simulink model "TailsitterSimModel_Trim"  (R2018b)
settings: Solver=ode23  StartTime=0  StopTime=1200  FixedStep=0.01  RelTol=1e-4  EnableMultiTasking=on
libraries: aerolibanimutils x1, tailsitter_lib x1, atmosphere_lib x1
settings Model: Creator=Yannic  LastModifiedBy=fabian
settings SolverCC: ZeroCrossControl=DisableAll  AlgebraicLoopSolver=LineSearch
settings DataIOCC: LimitDataPoints=on  SaveFormat=StructureWithTime
settings OptimizationCC: BlockReduction=off  DefaultParameterBehavior=Inlined  DefaultUnderspecifiedDataType=single  OptimizeBlockIOStorage=off  BufferReuse=off  GlobalBufferReuse=off  ExpressionFolding=off  LocalBlockOutputs=off  LifeSpan=inf  OptimizeDataStoreBuffers=off  BusAssignmentInplaceUpdate=off
settings DebuggingCC: AlgebraicLoopMsg=none  UnconnectedInputMsg=none  UnconnectedOutputMsg=none  UnconnectedLineMsg=none  AllowSymbolicDim=off  SFUnexpectedBacktrackingDiag=warning  SFNoUnconditionalDefaultTransitionDiag=warning  SFExecutionAtInitializationDiag=none
settings ModelReferenceCC: PropagateSignalLabelsOutOfModel=off
settings SFSimCC: SimUseLocalCustomCode=off
settings RTWCC: RTWUseLocalCustomCode=off
settings CodeAppCC: StateflowObjectComments=on
settings GRTTargetCC: TargetLangStandard=C89/C90 (ANSI)
settings ConfigComp: CovMetricSettings=dw  CovHtmlReporting=on  CovSaveCumulativeToWorkspaceVar=on  CovSaveSingleToWorkspaceVar=on  CovExternalEMLEnable=off

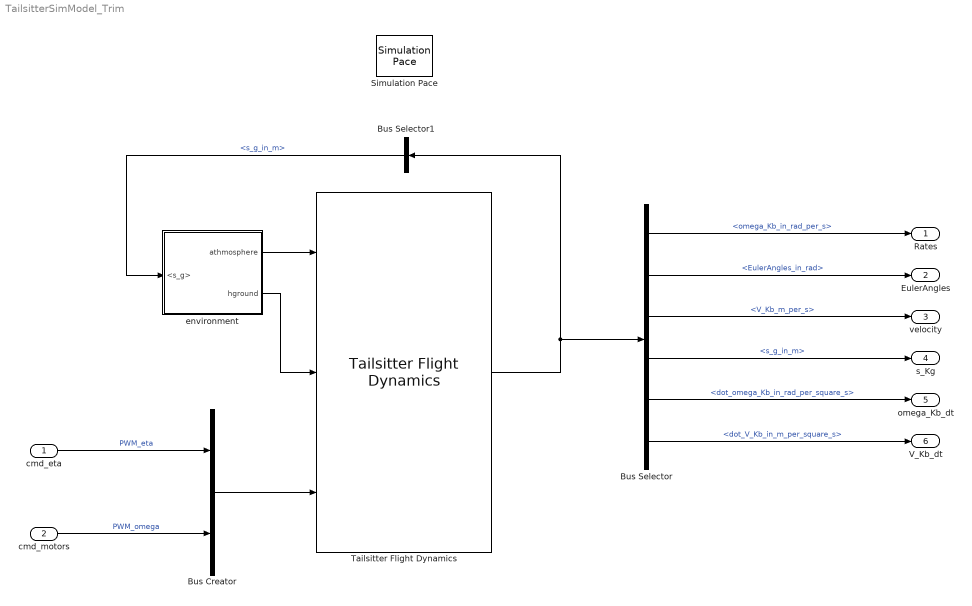
== system TailsitterSimModel_Trim ==
  cmd_eta : Inport  PortDimensions=2
  cmd_motors : Inport  Port=2  PortDimensions=2
  Bus Creator : BusCreator  Inputs=2
  Bus Selector : BusSelector  OutputSignals=rigid_body.omega_Kb_in_rad_per_s,rigid_body.EulerAngles_in_rad,rigid_body.V_Kb_m_per_s,rigid_body.s_g_in_m,rigid_body.dot_omega_Kb_in_rad_per_square_s,rigid_body.dot_V_Kb_in_m_per_square_s
  Bus Selector1 : BusSelector  OutputSignals=rigid_body.s_g_in_m
  Simulation Pace : aerolibanimutils/Simulation Pace  SimulationPace=pace  SleepMode=MATLAB Thread  OutputPaceError=off  SampleTime=1/30
  Tailsitter Flight Dynamics : tailsitter_lib/Tailsitter Flight Dynamics  tailsitter=tailsitter
      settings: SourceProductName=LADAC
  environment : Subsystem
  Rates : Outport
  EulerAngles : Outport  Port=2
  velocity : Outport  Port=3
  s_Kg : Outport  Port=4
  omega_Kb_dt : Outport  Port=5
  V_Kb_dt : Outport  Port=6
  wires:
  cmd_motors/1 -> Bus Creator/2  "PWM_omega"
  cmd_eta/1 -> Bus Creator/1  "PWM_eta"
  Bus Creator/1 -> Tailsitter Flight Dynamics/3
  Bus Selector/1 -> Rates/1  "<omega_Kb_in_rad_per_s>"
  Bus Selector/2 -> EulerAngles/1  "<EulerAngles_in_rad>"
  environment/1(athmosphere) -> Tailsitter Flight Dynamics/1
  environment/2(hground) -> Tailsitter Flight Dynamics/2
  Tailsitter Flight Dynamics/1 -> Bus Selector1/1, Bus Selector/1
  Bus Selector/4 -> s_Kg/1  "<s_g_in_m>"
  Bus Selector1/1 -> environment/1(<s_g>)  "<s_g_in_m>"
  Bus Selector/3 -> velocity/1  "<V_Kb_m_per_s>"
  Bus Selector/5 -> omega_Kb_dt/1  "<dot_omega_Kb_in_rad_per_square_s>"
  Bus Selector/6 -> V_Kb_dt/1  "<dot_V_Kb_in_m_per_square_s>"

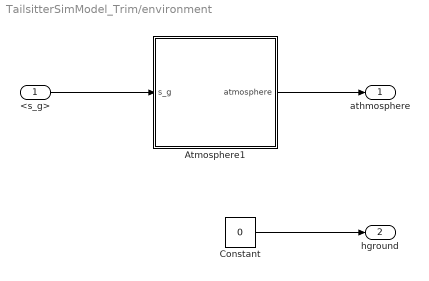
== system TailsitterSimModel_Trim/environment ==
  <s_g> : Inport
  Atmosphere1 : Subsystem
  Constant : Constant  Value=0
  athmosphere : Outport
  hground : Outport  Port=2
  wires:
  Constant/1 -> hground/1
  Atmosphere1/1(atmosphere) -> athmosphere/1
  <s_g>/1 -> Atmosphere1/1(s_g)

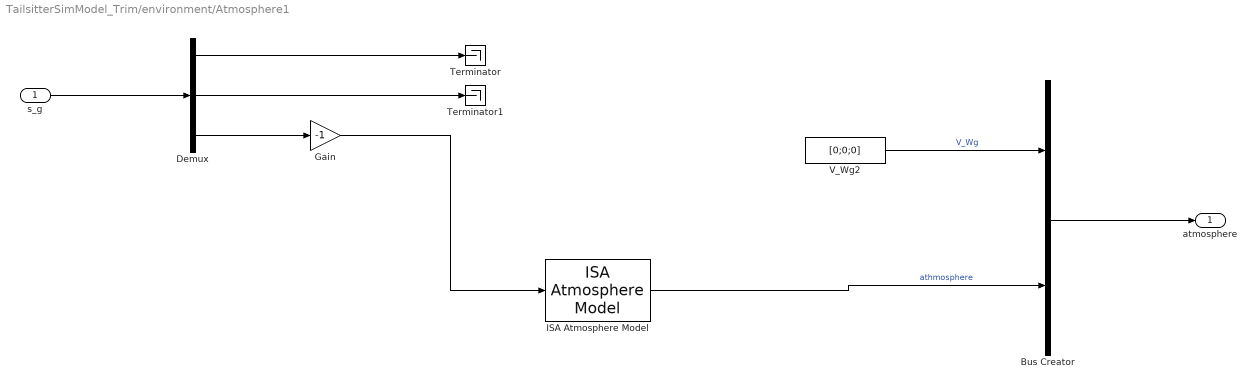
== system TailsitterSimModel_Trim/environment/Atmosphere1 ==
  s_g : Inport
  Bus Creator : BusCreator  Inputs=2
  Demux : Demux  Outputs=3
  Gain : Gain  Gain=-1
  ISA Atmosphere Model : atmosphere_lib/ISA Atmosphere Model  SystemSampleTime=-1
  Terminator : Terminator
  Terminator1 : Terminator
  V_Wg2 : Constant  Value=[0;0;0]
  atmosphere : Outport
  wires:
  ISA Atmosphere Model/1 -> Bus Creator/2  "athmosphere"
  Demux/1 -> Terminator/1
  Demux/2 -> Terminator1/1
  s_g/1 -> Demux/1
  Demux/3 -> Gain/1
  Gain/1 -> ISA Atmosphere Model/1
  Bus Creator/1 -> atmosphere/1
  V_Wg2/1 -> Bus Creator/1  "V_Wg"
